simulink model "FOC_Motor_Control"  (R2020b)
settings: Solver=FixedStepDiscrete  StartTime=0.0  StopTime=10.0  FixedStep=Fixed_Step_Size  RelTol=1e-3
values from neighbouring files (symbols this model uses):
  Angle = 1.0    [Hall_HSMO_FOC_Data.sldd]    (also in Hall_SMO_FOC_Data.sldd)
  Cosine_table = 1.0 0.99999529 0.99999058 0.99998587 0.99998116 0.99996704 0.99995291 0.99993885 0.99992472 0.99990118 0.99987763 0.99985409 0.9998306 0.99979764 0.99976468 0.99973178 0.99969882 0.99965644 0.99961412 0.99957174 0.99952942 0.99947762 0.99942589 0.99937415 0.99932235 0.9992612 0.99920005 0.99913889 0.99907768 0.99900717 0.99893659 0.99886602 0.99879545 0.99871546 0.99863547 0.99855554 0.99847555 0.    [Hall_HSMO_FOC_Data.sldd]    (also in Hall_SMO_FOC_Data.sldd)
  Flux = 0.0109    [G474_FOC_HSMO.sldd]    (also in Hall_HSMO_FOC_Data.sldd = 0.00529276
  HaLL_AngleShift = -0.25    [Hall_HSMO_FOC_Data.sldd]    (also in Hall_SMO_FOC_Data.sldd)
  HaLL_Sector1 = 5.236    [Hall_HSMO_FOC_Data.sldd]    (also in Hall_SMO_FOC_Data.sldd)
  HaLL_Sector2 = 1.0472    [Hall_HSMO_FOC_Data.sldd]    (also in Hall_SMO_FOC_Data.sldd)
  HaLL_Sector3 = 0.0    [Hall_HSMO_FOC_Data.sldd]    (also in Hall_SMO_FOC_Data.sldd)
  HaLL_Sector4 = 3.1415    [Hall_HSMO_FOC_Data.sldd]    (also in Hall_SMO_FOC_Data.sldd)
  HaLL_Sector5 = 4.1888    [Hall_HSMO_FOC_Data.sldd]    (also in Hall_SMO_FOC_Data.sldd)
  HaLL_Sector6 = 2.0944    [Hall_HSMO_FOC_Data.sldd]    (also in Hall_SMO_FOC_Data.sldd)
  HaLL_Timer_T = 1.0E-5    [Hall_HSMO_FOC_Data.sldd]    (also in Hall_SMO_FOC_Data.sldd)
  ID_Ki = 450.0    [Hall_HSMO_FOC_Data.sldd]    (also in Hall_SMO_FOC_Data.sldd = 0.8
  ID_Kp = 0.4    [Hall_HSMO_FOC_Data.sldd]    (also in Hall_SMO_FOC_Data.sldd = 3.2
  IQ_Ki = 450.0    [Hall_HSMO_FOC_Data.sldd]    (also in Hall_SMO_FOC_Data.sldd = 0.32
  IQ_Kp = 0.45    [Hall_HSMO_FOC_Data.sldd]    (also in Hall_SMO_FOC_Data.sldd = 3.3
  LADRC_b0 = 80000.0    [Hall_HSMO_FOC_Data.sldd]    (also in Hall_SMO_FOC_Data.sldd)
  LADRC_Omega_c = 80.0    [Hall_HSMO_FOC_Data.sldd]    (also in Hall_SMO_FOC_Data.sldd)
  Ld = 0.000195185    [G474_FOC_HSMO.sldd]    (also in Hall_HSMO_FOC_Data.sldd = 0.0004
  Lq = 0.000195185    [G474_FOC_HSMO.sldd]    (also in Hall_HSMO_FOC_Data.sldd = 0.00045
  OPL_Speed = 800.0    [Hall_HSMO_FOC_Data.sldd]
  OPL_Time = 5.0    [Hall_HSMO_FOC_Data.sldd]
  OPL_Torque = 3.0    [Hall_HSMO_FOC_Data.sldd]
  Over_modulation = 0.0    [Hall_HSMO_FOC_Data.sldd]    (also in Hall_SMO_FOC_Data.sldd)
  Pole_Pairs = 2.0    [Hall_HSMO_FOC_Data.sldd]    (also in Hall_SMO_FOC_Data.sldd)
  PWM_Frequency = 10000.0    [Hall_HSMO_FOC_Data.sldd]    (also in Hall_SMO_FOC_Data.sldd)
  R = 0.405    [Hall_HSMO_FOC_Data.sldd]    (also in Hall_SMO_FOC_Data.sldd = 0.4
  Sine_table = 0.0 0.0015339879 0.0030679768 0.0046019657 0.0061359555 0.0076698866 0.0092038177 0.010737749 0.012271681 0.013805497 0.015339312 0.016873131 0.018406944 0.019940587 0.021474229 0.023007872 0.024541514 0.026074925 0.027608337 0.029141748 0.03067516 0.032208283 0.033741407 0.035274528 0.036807653 0.038340431 0.039873205 0.04140598 0.042938754 0.04447113 0.046003502 0.047535874 0.049068246 0.0506001    [Hall_HSMO_FOC_Data.sldd]    (also in Hall_SMO_FOC_Data.sldd)
  SMO_K = 0.5    [Hall_HSMO_FOC_Data.sldd]    (also in Hall_SMO_FOC_Data.sldd)
  SMO_M = 0.15    [Hall_HSMO_FOC_Data.sldd]    (also in Hall_SMO_FOC_Data.sldd)
  SMO_PLL_W = 50.0    [Hall_HSMO_FOC_Data.sldd]    (also in Hall_SMO_FOC_Data.sldd)
  SMO_Theta_Enable = 0.0    [Hall_HSMO_FOC_Data.sldd]    (also in Hall_SMO_FOC_Data.sldd = 1.0
  Speed_Ki = 0.633    [Hall_HSMO_FOC_Data.sldd]    (also in Hall_SMO_FOC_Data.sldd)
  Speed_Kp = 0.0867    [Hall_HSMO_FOC_Data.sldd]    (also in Hall_SMO_FOC_Data.sldd = 0.0267
  Speed_PI_OutputMax = 6.0    [Hall_HSMO_FOC_Data.sldd]    (also in Hall_SMO_FOC_Data.sldd = 5.0
  Speed_PI_OutputMin = -6.0    [Hall_HSMO_FOC_Data.sldd]    (also in Hall_SMO_FOC_Data.sldd = -5.0
  SpeedFilter_Fn = 0.3    [Hall_HSMO_FOC_Data.sldd]    (also in Hall_SMO_FOC_Data.sldd)
  TorqueMode = 0.0    [Hall_HSMO_FOC_Data.sldd]    (also in Hall_SMO_FOC_Data.sldd)
undefined symbols (not defined in the file or in its folder): DiscIntNeverNeededParam, inverter, magnitude, SVPWM
libraries: simulink x6, pid_lib x1
(part 2 of 3)

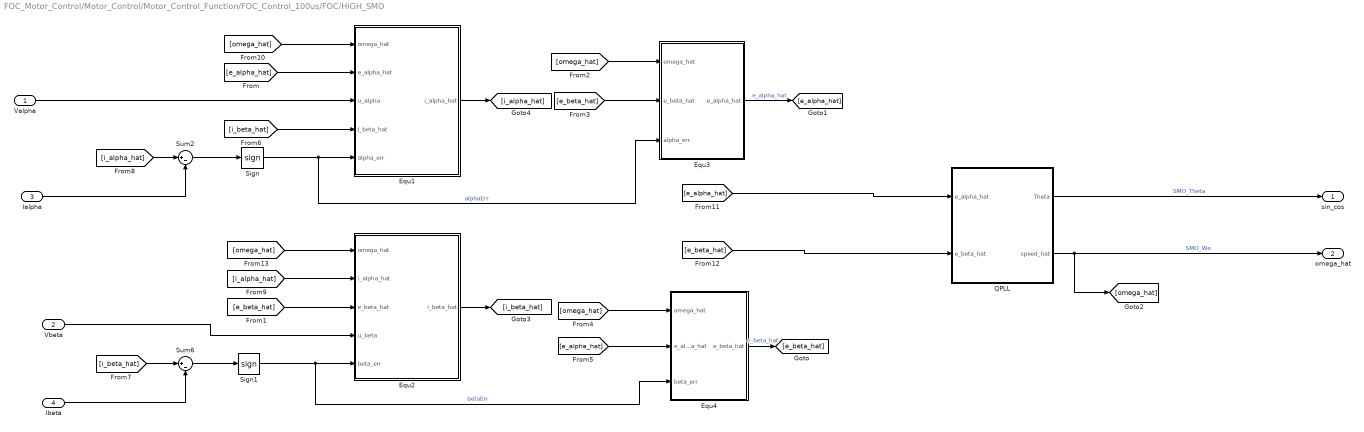
== system FOC_Motor_Control/Motor_Control/Motor_Control_Function/FOC_Control_100us/FOC/HIGH_SMO ==
  Valpha : Inport
  Vbeta : Inport  Port=2
  Ialpha : Inport  Port=3
  Ibeta : Inport  Port=4
  Equ1 : Subsystem
  Equ2 : Subsystem
  Equ3 : Subsystem
  Equ4 : Subsystem
  QPLL : Subsystem
  Sign : Signum
  Sign1 : Signum
  Sum2 : Sum  Inputs=|+-
  Sum6 : Sum  Inputs=|+-
  sin_cos : Outport
  omega_hat : Outport  Port=2
  wires:
  Sum6/1 -> Sign1/1
  Sum2/1 -> Sign/1
  Sign/1 -> Equ3/3(alpha_err), Equ1/5(alpha_err)  "alphaErr"
  Ialpha/1 -> Sum2/2
  Sign1/1 -> Equ4/3(beta_err), Equ2/5(beta_err)  "betaErr"
  Ibeta/1 -> Sum6/2
  Equ1/1(i_alpha_hat) -> [i_alpha_hat]
  [e_alpha_hat] -> Equ1/2(e_alpha_hat)
  Valpha/1 -> Equ1/3(u_alpha)
  [e_beta_hat] -> Equ2/3(e_beta_hat)
  Vbeta/1 -> Equ2/4(u_beta)
  Equ2/1(i_beta_hat) -> [i_beta_hat]
  [i_beta_hat] -> Equ1/4(I_beta_hat)
  [i_beta_hat] -> Sum6/1
  [i_alpha_hat] -> Sum2/1
  [i_alpha_hat] -> Equ2/2(i_alpha_hat)
  [omega_hat] -> Equ3/1(omega_hat)
  [e_beta_hat] -> Equ3/2(e_beta_hat)
  [omega_hat] -> Equ4/1(omega_hat)
  [e_alpha_hat] -> Equ4/2(e_alpha_hat)
  [omega_hat] -> Equ1/1(omega_hat)
  Equ4/1(e_beta_hat) -> [e_beta_hat]  "e_beta_hat"
  Equ3/1(e_alpha_hat) -> [e_alpha_hat]  "e_alpha_hat"
  [e_alpha_hat] -> QPLL/1(e_alpha_hat)
  [e_beta_hat] -> QPLL/2(e_beta_hat)
  QPLL/2(speed_hat) -> [omega_hat], omega_hat/1  "SMO_We"
  QPLL/1(Theta) -> sin_cos/1  "SMO_Theta"
  [omega_hat] -> Equ2/1(omega_hat)

== system FOC_Motor_Control/Motor_Control/Motor_Control_Function/FOC_Control_100us/FOC/Hall_Angle ==
  Hall_Angle : Inport
  Action Port : ActionPort  ActionPortLabel=elseif(u1==0)
  Out1 : Outport
  wires:
  Hall_Angle/1 -> Out1/1

== system FOC_Motor_Control/Motor_Control/Motor_Control_Function/FOC_Control_100us/FOC/Inverse_Park_Transform ==
  D : Inport
  Q : Inport  Port=2
  Sin_Coefficient : Inport  Port=3
  Cos_Coefficient : Inport  Port=4
  Add1 : Sum  Inputs=+-  OutDataTypeStr=Inherit: Same as first input
  Add2 : Sum  OutDataTypeStr=Inherit: Same as first input
  Cos_Coefficient1 : InportShadow  Port=4
  Product{1..4} (4 alike) : Product  RndMeth=Simplest  OutDataTypeStr=Inherit: Same as first input
  Sin_Coefficient1 : InportShadow  Port=3
  Alpha : Outport  VectorParamsAs1DForOutWhenUnconnected=off
  Beta : Outport  Port=2  VectorParamsAs1DForOutWhenUnconnected=off
  wires:
  Product3/1 -> Add2/1
  Product4/1 -> Add2/2
  Product1/1 -> Add1/1
  Product2/1 -> Add1/2
  Cos_Coefficient1/1 -> Product4/2
  Sin_Coefficient/1 -> Product2/2
  D/1 -> Product3/1, Product1/1
  Q/1 -> Product2/1, Product4/1
  Sin_Coefficient1/1 -> Product3/2
  Cos_Coefficient/1 -> Product1/2
  Add1/1 -> Alpha/1
  Add2/1 -> Beta/1

== system FOC_Motor_Control/Motor_Control/Motor_Control_Function/FOC_Control_100us/FOC/LPF ==
  u : Inport
  Add : Sum  Inputs=+-
  Add1 : Sum
  Constant1 : Constant  Value=SpeedFilter_Fn  OutDataTypeStr=single
  Divide1 : Product  Inputs=**
  Unit Delay : UnitDelay  SampleTime=-1  HasFrameUpgradeWarning=on
  y : Outport
  wires:
  Constant1/1 -> Divide1/1
  u/1 -> Add/1
  Add/1 -> Divide1/2
  Divide1/1 -> Add1/1
  Unit Delay/1 -> Add/2, Add1/2
  Add1/1 -> Unit Delay/1, y/1

== system FOC_Motor_Control/Motor_Control/Motor_Control_Function/FOC_Control_100us/FOC/Obs_Angle ==
  Obs_Angle : Inport
  Action Port : ActionPort  ActionPortLabel=if(u1==1)
  Out1 : Outport
  wires:
  Obs_Angle/1 -> Out1/1

== system FOC_Motor_Control/Motor_Control/Motor_Control_Function/FOC_Control_100us/FOC/OpenLoop ==
  OPL_Speed : Inport
  OPL_Torque : Inport  Port=2
  OPL_Time : Inport  Port=3
  Action Port : ActionPort  ActionPortLabel=case [ 1 ]:
  2pi2 : Constant  Value=2*pi  OutDataTypeStr=single
  Discrete-Time Integrator1 : DiscreteIntegrator  SampleTime=-1  ICPrevOutput=DiscIntNeverNeededParam  ICPrevScaledInput=DiscIntNeverNeededParam
  Discrete-Time Integrator2 : DiscreteIntegrator  SampleTime=-1  ICPrevOutput=DiscIntNeverNeededParam  ICPrevScaledInput=DiscIntNeverNeededParam
  Mod2 : Math  Operator=mod  SaturateOnIntegerOverflow=on
  Product : Product
  Scope : Scope
  Scope1 : Scope
  We : Gain  Gain=Pole_Pairs*2*pi/60  OutDataTypeStr=single  ParamDataTypeStr=Inherit: Same as input
  Force_Angle : Outport
  OPL_Torque_Com : Outport  Port=2
  wires:
  OPL_Speed/1 -> Product/1
  Product/1 -> Discrete-Time Integrator2/1
  Discrete-Time Integrator1/1 -> Mod2/1
  Discrete-Time Integrator2/1 -> Scope/1, We/1
  We/1 -> Discrete-Time Integrator1/1  "Delta_Theta"
  Mod2/1 -> Force_Angle/1, Scope1/1
  OPL_Torque/1 -> OPL_Torque_Com/1
  OPL_Time/1 -> Product/2
  2pi2/1 -> Mod2/2

== system FOC_Motor_Control/Motor_Control/Motor_Control_Function/FOC_Control_100us/FOC/Park_Transform ==
  Alpha : Inport
  Beta : Inport  Port=2
  Sin_Coefficient : Inport  Port=3
  Cos_Coefficient : Inport  Port=4
  Add1 : Sum  OutDataTypeStr=Inherit: Same as first input
  Add2 : Sum  Inputs=-+  OutDataTypeStr=Inherit: Same as first input
  Alpha1 : InportShadow
  Beta1 : InportShadow  Port=2
  Cos_Coefficient1 : InportShadow  Port=4
  Produc3t : Product  RndMeth=Simplest  OutDataTypeStr=Inherit: Same as first input
  Product1 : Product  RndMeth=Simplest  OutDataTypeStr=Inherit: Same as first input
  Product2 : Product  RndMeth=Simplest  OutDataTypeStr=Inherit: Same as first input
  Product4 : Product  RndMeth=Simplest  OutDataTypeStr=Inherit: Same as first input
  Sin_Coefficient1 : InportShadow  Port=3
  D : Outport  VectorParamsAs1DForOutWhenUnconnected=off
  Q : Outport  Port=2  VectorParamsAs1DForOutWhenUnconnected=off
  wires:
  Produc3t/1 -> Add2/1
  Product4/1 -> Add2/2
  Product1/1 -> Add1/1
  Product2/1 -> Add1/2
  Alpha1/1 -> Produc3t/1
  Sin_Coefficient1/1 -> Produc3t/2
  Cos_Coefficient1/1 -> Product4/2
  Beta1/1 -> Product4/1
  Alpha/1 -> Product1/1
  Cos_Coefficient/1 -> Product1/2
  Beta/1 -> Product2/1
  Sin_Coefficient/1 -> Product2/2
  Add1/1 -> D/1
  Add2/1 -> Q/1

== system FOC_Motor_Control/Motor_Control/Motor_Control_Function/FOC_Control_100us/FOC/Q_Current_PI ==
  Reset : Inport
  Bus_voltage : Inport  Port=2
  Current_Command : Inport  Port=3
  Current_Measured : Inport  Port=4
  Add2 : Sum  Inputs=|+-
  IQ_Control : Subsystem
  Vq_voltage : Outport  VectorParamsAs1DForOutWhenUnconnected=off
  wires:
  Current_Command/1 -> Add2/1
  Current_Measured/1 -> Add2/2
  Add2/1 -> IQ_Control/3(Err)  "currentControlError"
  Reset/1 -> IQ_Control/1(Reset)
  Bus_voltage/1 -> IQ_Control/2(Bus_voltage)
  IQ_Control/1(PI_Out) -> Vq_voltage/1

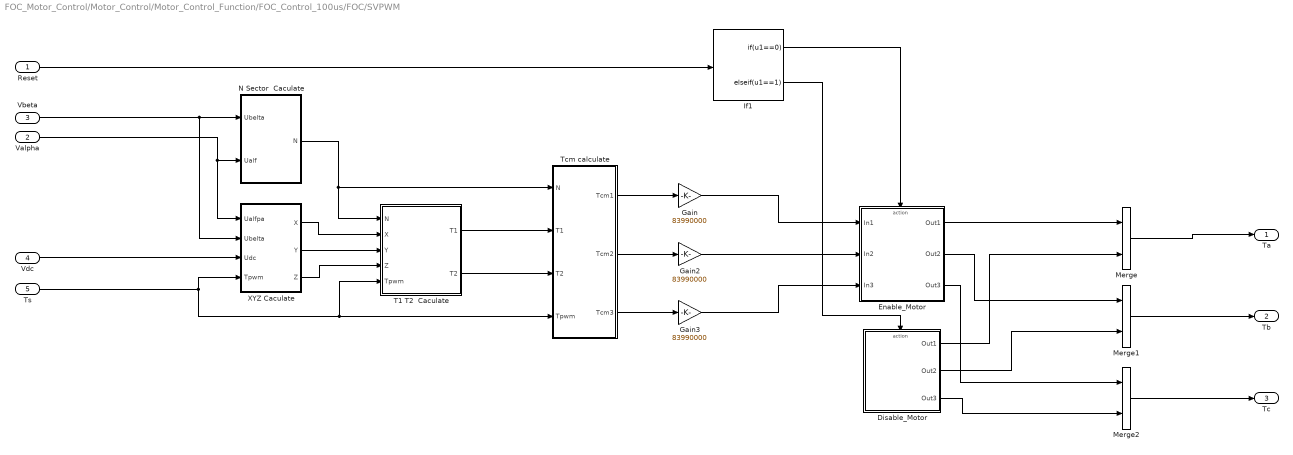
== system FOC_Motor_Control/Motor_Control/Motor_Control_Function/FOC_Control_100us/FOC/SVPWM ==
  Reset : Inport
  Valpha : Inport  Port=2
  Vbeta : Inport  Port=3
  Vdc : Inport  Port=4
  Ts : Inport  Port=5
  Disable_Motor : Subsystem  TreatAsAtomicUnit=on
  Enable_Motor : Subsystem  TreatAsAtomicUnit=on
  Gain : Gain  Gain=83990000
  Gain2 : Gain  Gain=83990000
  Gain3 : Gain  Gain=83990000
  If1 : If  IfExpression=u1==0  ElseIfExpressions=u1==1  ShowElse=off
  Merge : Merge
  Merge1 : Merge
  Merge2 : Merge
  N Sector  Caculate : Subsystem  TreatAsAtomicUnit=on
  T1 T2  Caculate : Subsystem  TreatAsAtomicUnit=on
  Tcm calculate : Subsystem  TreatAsAtomicUnit=on
  XYZ Caculate : Subsystem  TreatAsAtomicUnit=on
  Ta : Outport
  Tb : Outport  Port=2
  Tc : Outport  Port=3
  wires:
  T1 T2  Caculate/2(T2) -> Tcm calculate/3(T2)
  XYZ Caculate/1(X) -> T1 T2  Caculate/2(X)
  N Sector  Caculate/1(N) -> T1 T2  Caculate/1(N), Tcm calculate/1(N)
  Vdc/1 -> XYZ Caculate/3(Udc)
  T1 T2  Caculate/1(T1) -> Tcm calculate/2(T1)
  XYZ Caculate/3(Z) -> T1 T2  Caculate/4(Z)
  XYZ Caculate/2(Y) -> T1 T2  Caculate/3(Y)
  Valpha/1 -> N Sector  Caculate/2(Ualf), XYZ Caculate/1(Ualfpa)
  Vbeta/1 -> N Sector  Caculate/1(Ubelta), XYZ Caculate/2(Ubelta)
  Ts/1 -> T1 T2  Caculate/5(Tpwm), Tcm calculate/4(Tpwm), XYZ Caculate/4(Tpwm)
  Gain/1 -> Enable_Motor/1(In1)
  Gain2/1 -> Enable_Motor/2(In2)
  Reset/1 -> If1/1
  If1/1 -> Enable_Motor/Action
  If1/2 -> Disable_Motor/Action
  Gain3/1 -> Enable_Motor/3(In3)
  Enable_Motor/1(Out1) -> Merge/1
  Disable_Motor/1(Out1) -> Merge/2
  Enable_Motor/2(Out2) -> Merge1/1
  Disable_Motor/2(Out2) -> Merge1/2
  Enable_Motor/3(Out3) -> Merge2/1
  Disable_Motor/3(Out3) -> Merge2/2
  Merge/1 -> Ta/1
  Merge1/1 -> Tb/1
  Merge2/1 -> Tc/1
  Tcm calculate/1(Tcm1) -> Gain/1
  Tcm calculate/2(Tcm2) -> Gain2/1
  Tcm calculate/3(Tcm3) -> Gain3/1

== system FOC_Motor_Control/Motor_Control/Motor_Control_Function/FOC_Control_100us/FOC/Sine_Cosine ==
  note: Sine Cosine Coefficients
  P : Inport
  Cosine : Lookup_n-D  NumberOfTableDimensions=1  LookupTableObject=''  BreakpointsForDimension1=[0:2*pi/4095:2*pi]  BreakpointsForDimension1FirstPoint=10  BreakpointsForDimension2FirstPoint=10  BreakpointsForDimension1Spacing=12  BreakpointsForDimension2Spacing=12  IndexSearchMethod=Evenly spaced points  Table=Cosine_table  InterpMethod=Flat  DiagnosticForOutOfRangeInput=Error  InternalRulePriority=Speed  RndMeth=Simplest  InputSameDT=on
  Saturation : Saturate  UpperLimit=2*pi-0.0001  LowerLimit=0+0.0001
  Scope : Scope  NumInputPorts=2
  Sine : Lookup_n-D  NumberOfTableDimensions=1  LookupTableObject=''  BreakpointsForDimension1=[0:2*pi/4095:2*pi]  BreakpointsForDimension1FirstPoint=10  BreakpointsForDimension2FirstPoint=10  BreakpointsForDimension1Spacing=12  BreakpointsForDimension2Spacing=12  IndexSearchMethod=Evenly spaced points  Table=Sine_table  InterpMethod=Flat  DiagnosticForOutOfRangeInput=Error  InternalRulePriority=Speed  RndMeth=Simplest  InputSameDT=on
  Sin : Outport  VectorParamsAs1DForOutWhenUnconnected=off
  Cos : Outport  Port=2  VectorParamsAs1DForOutWhenUnconnected=off
  wires:
  P/1 -> Saturation/1  "position"
  Sine/1 -> Scope/1, Sin/1
  Cosine/1 -> Scope/2, Cos/1
  Saturation/1 -> Cosine/1, Sine/1

== system FOC_Motor_Control/Motor_Control/Motor_Control_Function/FOC_Control_100us/FOC/Subsystem ==
  In1 : Inport
  In2 : Inport  Port=2
  Action Port : ActionPort  ActionPortLabel=case [ 2 ]:
  Out1 : Outport
  Out2 : Outport  Port=2
  wires:
  In1/1 -> Out1/1
  In2/1 -> Out2/1

== system FOC_Motor_Control/Motor_Control/Motor_Control_Function/Angle_Speed_100us/SpeedAndAngle/ACC_OMG/LPF ==
  u : Inport
  Add : Sum  Inputs=+-
  Add1 : Sum
  Constant1 : Constant  Value=SpeedFilter_Fn  OutDataTypeStr=single
  Divide1 : Product  Inputs=**
  Unit Delay : UnitDelay  SampleTime=-1  HasFrameUpgradeWarning=on
  y : Outport
  wires:
  Constant1/1 -> Divide1/1
  u/1 -> Add/1
  Add/1 -> Divide1/2
  Divide1/1 -> Add1/1
  Unit Delay/1 -> Add/2, Add1/2
  Add1/1 -> Unit Delay/1, y/1

== system FOC_Motor_Control/Motor_Control/Motor_Control_Function/Angle_Speed_100us/SpeedAndAngle/ACC_OMG/Six_point ==
  In1 : Inport
  Merge2 : Merge  Inputs=6
  Scope : Scope  NumInputPorts=2
  Sector_1 : Subsystem
  Sector_2 : Subsystem
  Sector_3 : Subsystem
  Sector_4 : Subsystem
  Sector_5 : Subsystem
  Sector_6 : Subsystem
  Switch Case2 : SwitchCase  CaseConditions={1,2,3,4,5,6}  ShowDefaultCase=off
  Out1 : Outport
  wires:
  Sector_4/1(Angle_0) -> Merge2/4
  Switch Case2/5 -> Sector_5/Action
  Sector_6/1(Angle_0) -> Merge2/6
  Sector_5/1(Angle_0) -> Merge2/5
  Switch Case2/6 -> Sector_6/Action
  Switch Case2/3 -> Sector_3/Action
  Switch Case2/4 -> Sector_4/Action
  Sector_1/1(Angle_0) -> Merge2/1
  Switch Case2/2 -> Sector_2/Action
  In1/1 -> Scope/1, Switch Case2/1
  Sector_3/1(Angle_0) -> Merge2/3
  Switch Case2/1 -> Sector_1/Action
  Sector_2/1(Angle_0) -> Merge2/2
  Merge2/1 -> Scope/2, Out1/1

== system FOC_Motor_Control/Motor_Control/Motor_Control_Function/Angle_Speed_100us/SpeedAndAngle/ADC_IRQ/HallAngle_calibration ==
  Angle_input : Inport
  Angle_offset : Constant  Value=HaLL_AngleShift
  If Action Subsystem1 : Subsystem  TreatAsAtomicUnit=on
  If Action Subsystem2 : Subsystem  TreatAsAtomicUnit=on
  If Action Subsystem3 : Subsystem  TreatAsAtomicUnit=on
  If1 : If  IfExpression=u1 > 6.283185307  ElseIfExpressions=u1<0
  Merge1 : Merge  Inputs=3
  Subtract1 : Sum
  Angle_output : Outport
  wires:
  Angle_input/1 -> Subtract1/1
  Angle_offset/1 -> Subtract1/2  "Control_ModeCommand"
  If1/1 -> If Action Subsystem2/Action
  If1/3 -> If Action Subsystem1/Action
  If Action Subsystem2/1(Out1) -> Merge1/1
  Subtract1/1 -> If Action Subsystem3/1(In1), If Action Subsystem1/1(In1), If Action Subsystem2/1(In1), If1/1
  If Action Subsystem1/1(Out1) -> Merge1/3
  If Action Subsystem3/1(Out1) -> Merge1/2
  If1/2 -> If Action Subsystem3/Action
  Merge1/1 -> Angle_output/1

== system FOC_Motor_Control/Motor_Control/Motor_Control_Function/Angle_Speed_100us/Speed_Resolver/Speed_cacl/LPF ==
  u : Inport
  Add : Sum  Inputs=+-
  Add1 : Sum
  Constant1 : Constant  Value=SpeedFilter_Fn  OutDataTypeStr=single
  Divide1 : Product  Inputs=**
  Unit Delay : UnitDelay  SampleTime=-1  HasFrameUpgradeWarning=on
  y : Outport
  wires:
  Constant1/1 -> Divide1/1
  u/1 -> Add/1
  Add/1 -> Divide1/2
  Divide1/1 -> Add1/1
  Unit Delay/1 -> Add/2, Add1/2
  Add1/1 -> Unit Delay/1, y/1

== system FOC_Motor_Control/Motor_Control/Motor_Control_Function/Control_Command_2ms/Control_Command_2ms/Speed_PI/SpeedLoop ==
  CMD_RPM : Inport  OutDataTypeStr=single
  FdkRPM : Inport  Port=2  OutDataTypeStr=single
  Reset : Inport  Port=3
  Constant : Constant  Value=LADRC_b0  OutDataTypeStr=single  SampleTime=-1
  Divide : Product  Inputs=*/  OutDataTypeStr=single
  LESO : Subsystem
  Saturation : Saturate  UpperLimit=Speed_PI_OutputMax  LowerLimit=Speed_PI_OutputMin  OutDataTypeStr=single
  Sum : Sum  Inputs=|+-  OutDataTypeStr=single
  Sum1 : Sum  Inputs=|+-  OutDataTypeStr=single
  Unit Delay : UnitDelay  SampleTime=-1  HasFrameUpgradeWarning=on
  omega_c : Gain  Gain=LADRC_Omega_c  OutDataTypeStr=single
  RefIq : Outport  OutDataTypeStr=single
  wires:
  Saturation/1 -> RefIq/1, Unit Delay/1
  Constant/1 -> Divide/2
  Divide/1 -> Saturation/1
  LESO/2(f_hat) -> Sum1/2
  FdkRPM/1 -> LESO/1(FbkSpd)  "FdkRPM"
  LESO/1(omega_r_hat) -> Sum/2
  Sum1/1 -> Divide/1
  omega_c/1 -> Sum1/1
  Sum/1 -> omega_c/1
  CMD_RPM/1 -> Sum/1  "CMD_RPM"
  Unit Delay/1 -> LESO/2(iq)
  Reset/1 -> LESO/3(Reset)

== system FOC_Motor_Control/Motor_Control/Motor_Control_Function/Control_Command_2ms/Control_Command_2ms/Speed_PI/Speed_PI ==
  Ref : Inport
  Fdk : Inport  Port=2
  Reset : Inport  Port=3
  Speed_Control : Subsystem
  Sum : Sum  Inputs=|+-
  PI_out : Outport  VectorParamsAs1DForOutWhenUnconnected=off
  wires:
  Speed_Control/1(PI_Out) -> PI_out/1
  Reset/1 -> Speed_Control/2(Reset)
  Ref/1 -> Sum/1
  Sum/1 -> Speed_Control/1(Err)
  Fdk/1 -> Sum/2

== system FOC_Motor_Control/Motor_Control/Motor_Control_Function/FOC_Control_100us/FOC/Clarke_Transform/Clark1 ==
  Iabc : Inport
  Add : Sum  Inputs=+--
  Add1 : Sum  Inputs=+-
  Demux : Demux  Outputs=3
  Gain : Gain  Gain=0.5
  Gain1 : Gain  Gain=0.5
  Gain2 : Gain  Gain=sqrt(2/3)
  Gain3 : Gain  Gain=sqrt(3)/2
  Gain4 : Gain  Gain=sqrt(3)/2
  Gain5 : Gain  Gain=sqrt(2/3)
  Ialpha : Outport  VectorParamsAs1DForOutWhenUnconnected=off
  Ibeta : Outport  Port=2  VectorParamsAs1DForOutWhenUnconnected=off
  wires:
  Iabc/1 -> Demux/1
  Demux/1 -> Add/1
  Gain/1 -> Add/2
  Demux/2 -> Gain3/1, Gain/1
  Gain1/1 -> Add/3
  Demux/3 -> Gain4/1, Gain1/1
  Add/1 -> Gain2/1
  Gain2/1 -> Ialpha/1
  Gain3/1 -> Add1/1
  Gain4/1 -> Add1/2
  Add1/1 -> Gain5/1
  Gain5/1 -> Ibeta/1

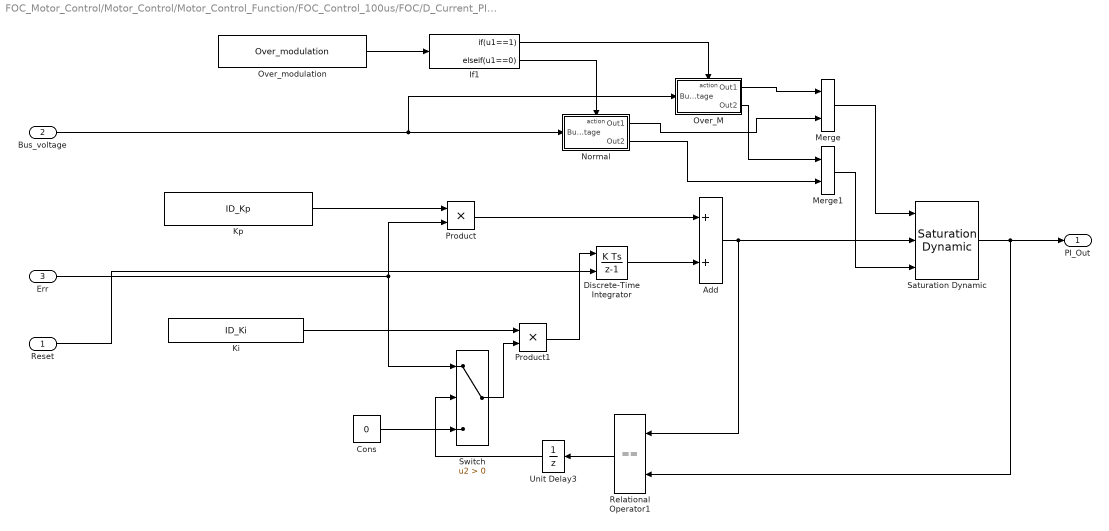
== system FOC_Motor_Control/Motor_Control/Motor_Control_Function/FOC_Control_100us/FOC/D_Current_PI/ID_Control ==
  Reset : Inport
  Bus_voltage : Inport  Port=2
  Err : Inport  Port=3
  Add : Sum
  Cons : Constant  Value=0  OutDataTypeStr=single
  Discrete-Time Integrator : DiscreteIntegrator  ExternalReset=level  SampleTime=-1  ICPrevOutput=DiscIntNeverNeededParam  ICPrevScaledInput=DiscIntNeverNeededParam
  If1 : If  IfExpression=u1==1  ElseIfExpressions=u1==0  ShowElse=off
  Ki : Constant  Value=ID_Ki  OutDataTypeStr=single
  Kp : Constant  Value=ID_Kp  OutDataTypeStr=single
  Merge : Merge
  Merge1 : Merge
  Normal : Subsystem  TreatAsAtomicUnit=on
  Over_M : Subsystem  TreatAsAtomicUnit=on
  Over_modulation : Constant  Value=Over_modulation  OutDataTypeStr=boolean
  Product : Product
  Product1 : Product
  Relational Operator1 : RelationalOperator  Operator===  OutDataTypeStr=boolean  RndMeth=Simplest
  Saturation Dynamic : simulink/Discontinuities/Saturation Dynamic  OutMin=[]  OutMax=[]  OutDataTypeStr=Inherit: Same as second input  OutDataType=fixdt(1, 16)  OutScaling=2^-10  DoSatur=off
  Switch : Switch  Criteria=u2 > Threshold
  Unit Delay3 : UnitDelay  SampleTime=-1  HasFrameUpgradeWarning=on
  PI_Out : Outport
  wires:
  Kp/1 -> Product/1
  Err/1 -> Product/2, Switch/1
  Switch/1 -> Product1/2
  Product1/1 -> Discrete-Time Integrator/1
  Product/1 -> Add/1
  Add/1 -> Saturation Dynamic/2, Relational Operator1/1
  Saturation Dynamic/1 -> Relational Operator1/2, PI_Out/1
  Cons/1 -> Switch/3
  Discrete-Time Integrator/1 -> Add/2
  Relational Operator1/1 -> Unit Delay3/1
  Ki/1 -> Product1/1
  Unit Delay3/1 -> Switch/2
  Reset/1 -> Discrete-Time Integrator/2
  Over_modulation/1 -> If1/1
  If1/2 -> Normal/Action
  If1/1 -> Over_M/Action
  Bus_voltage/1 -> Over_M/1(Bus_voltage), Normal/1(Bus_voltage)
  Over_M/1(Out1) -> Merge/1
  Normal/1(Out1) -> Merge/2
  Over_M/2(Out2) -> Merge1/1
  Normal/2(Out2) -> Merge1/2
  Merge/1 -> Saturation Dynamic/1
  Merge1/1 -> Saturation Dynamic/3

== system FOC_Motor_Control/Motor_Control/Motor_Control_Function/FOC_Control_100us/FOC/HIGH_SMO/Equ1 ==
  note: GainK/Ld
  note: R/Ld
  note: (Ld-Lq)/Ld
  note: 1/Ld
  note: 1/Ld
  omega_hat : Inport
  e_alpha_hat : Inport  Port=2
  u_alpha : Inport  Port=3
  I_beta_hat : Inport  Port=4
  alpha_err : Inport  Port=5
  Add : Sum  Inputs=---+-
  Gain : Gain  Gain=R/Ld
  Gain1 : Gain  Gain=(Ld-Lq)/Ld
  Gain17 : Gain  Gain=1/Ld
  Gain2 : Gain  Gain=1/Ld
  Gain4 : Gain  Gain=SMO_K/Ld
  Integrator : DiscreteIntegrator  IntegratorMethod=Integration: Backward Euler  SampleTime=-1  ICPrevOutput=DiscIntNeverNeededParam  ICPrevScaledInput=DiscIntNeverNeededParam  mask(DiscretizedDiscreteIntegrator){}
      mask init:
      | %tustin
  Product : Product
  Unit Delay : UnitDelay  SampleTime=-1  HasFrameUpgradeWarning=on
  i_alpha_hat : Outport
  wires:
  Gain1/1 -> Add/2
  Gain4/1 -> Add/5
  Product/1 -> Gain1/1
  Add/1 -> Integrator/1
  I_beta_hat/1 -> Product/1
  Unit Delay/1 -> [i_alpha_hat], i_alpha_hat/1
  Gain/1 -> Add/1
  u_alpha/1 -> Gain2/1
  Gain2/1 -> Add/4
  Integrator/1 -> Unit Delay/1
  omega_hat/1 -> Product/2
  Gain17/1 -> Add/3
  e_alpha_hat/1 -> Gain17/1
  alpha_err/1 -> Gain4/1
  [i_alpha_hat] -> Gain/1

== system FOC_Motor_Control/Motor_Control/Motor_Control_Function/FOC_Control_100us/FOC/HIGH_SMO/Equ2 ==
  note: R/Ld
  note: (Ld-Lq)/Ld
  note: 1/Ld
  note: 1/Ld
  note: GainK/Ld
  omega_hat : Inport
  i_alpha_hat : Inport  Port=2
  e_beta_hat : Inport  Port=3
  u_beta : Inport  Port=4
  beta_err : Inport  Port=5
  Add1 : Sum  Inputs=+--+-
  Gain3 : Gain  Gain=1/Ld
  Gain5 : Gain  Gain=1/Ld
  Gain6 : Gain  Gain=SMO_K/Ld
  Gain7 : Gain  Gain=(Ld-Lq)/Ld
  Gain8 : Gain  Gain=R/Ld
  Integrator1 : DiscreteIntegrator  IntegratorMethod=Integration: Backward Euler  SampleTime=-1  ICPrevOutput=DiscIntNeverNeededParam  ICPrevScaledInput=DiscIntNeverNeededParam  mask(DiscretizedDiscreteIntegrator){}
      mask init:
      | %tustin
  Product1 : Product
  Unit Delay1 : UnitDelay  SampleTime=-1  HasFrameUpgradeWarning=on
  i_beta_hat : Outport
  wires:
  Gain8/1 -> Add1/2
  u_beta/1 -> Gain5/1
  Add1/1 -> Integrator1/1
  Gain3/1 -> Add1/3
  i_alpha_hat/1 -> Product1/1
  Gain5/1 -> Add1/4
  Gain6/1 -> Add1/5
  Integrator1/1 -> Unit Delay1/1
  Product1/1 -> Gain7/1
  Gain7/1 -> Add1/1
  beta_err/1 -> Gain6/1
  e_beta_hat/1 -> Gain3/1
  Unit Delay1/1 -> [I_beta_hat], i_beta_hat/1
  omega_hat/1 -> Product1/2
  [I_beta_hat] -> Gain8/1

== system FOC_Motor_Control/Motor_Control/Motor_Control_Function/FOC_Control_100us/FOC/HIGH_SMO/Equ3 ==
  omega_hat : Inport
  e_beta_hat : Inport  Port=2
  alpha_err : Inport  Port=3
  Add2 : Sum  Inputs=-+
  Gain9 : Gain  Gain=SMO_M/Ld
  Integrator2 : DiscreteIntegrator  IntegratorMethod=Integration: Backward Euler  SampleTime=-1  ICPrevOutput=DiscIntNeverNeededParam  ICPrevScaledInput=DiscIntNeverNeededParam  mask(DiscretizedDiscreteIntegrator){}
      mask init:
      | %tustin
  Product2 : Product
  Unit Delay2 : UnitDelay  SampleTime=-1  HasFrameUpgradeWarning=on
  e_alpha_hat : Outport
  wires:
  alpha_err/1 -> Gain9/1
  Add2/1 -> Integrator2/1
  Unit Delay2/1 -> e_alpha_hat/1
  omega_hat/1 -> Product2/1
  Product2/1 -> Add2/1
  Integrator2/1 -> Unit Delay2/1
  e_beta_hat/1 -> Product2/2
  Gain9/1 -> Add2/2

== system FOC_Motor_Control/Motor_Control/Motor_Control_Function/FOC_Control_100us/FOC/HIGH_SMO/Equ4 ==
  omega_hat : Inport
  e_alpha_hat : Inport  Port=2
  beta_err : Inport  Port=3
  Add3 : Sum
  Gain10 : Gain  Gain=SMO_K/Ld
  Integrator3 : DiscreteIntegrator  IntegratorMethod=Integration: Backward Euler  SampleTime=-1  ICPrevOutput=DiscIntNeverNeededParam  ICPrevScaledInput=DiscIntNeverNeededParam  mask(DiscretizedDiscreteIntegrator){}
      mask init:
      | %tustin
  Product3 : Product
  Unit Delay3 : UnitDelay  SampleTime=-1  HasFrameUpgradeWarning=on
  e_beta_hat : Outport
  wires:
  Integrator3/1 -> Unit Delay3/1
  Add3/1 -> Integrator3/1
  Gain10/1 -> Add3/2
  Product3/1 -> Add3/1
  beta_err/1 -> Gain10/1
  Unit Delay3/1 -> e_beta_hat/1
  omega_hat/1 -> Product3/1
  e_alpha_hat/1 -> Product3/2

== system FOC_Motor_Control/Motor_Control/Motor_Control_Function/FOC_Control_100us/FOC/HIGH_SMO/QPLL ==
  e_alpha_hat : Inport
  e_beta_hat : Inport  Port=2
  Ki : Constant  Value=SMO_PLL_W*SMO_PLL_W  OutDataTypeStr=single
  Kp : Constant  Value=2*0.707*SMO_PLL_W  OutDataTypeStr=single
  PIDTheta_Ctrl : pid_lib/PID Controller  Controller=PI  Form=Parallel  TimeDomain=Discrete-time  UseExternalTs=off  SampleTime=-1  IntegratorMethod=Forward Euler  FilterMethod=Forward Euler  ControllerParametersSource=external  P=2*0.707*SMO_PLL_W  I=SMO_PLL_W*SMO_PLL_W  D=0  UseFilter=on  N=100  TunerSelectOption=Transfer Function Based (PID Tuner App)  ZeroCross=off  InitialConditionSource=internal  InitialConditionForIntegrator=1  InitialConditionForFilter=0  DifferentiatorICPrevScaledInput=0  ExternalReset=none  TrackingMode=off  Kt=1  LimitOutput=on  SatLimitsSource=internal  UpperSaturationLimit=2*pi*500  LowerSaturationLimit=-2*pi*500  LinearizeAsGain=off  AntiWindupMode=clamping  Kb=50  POutMin=[]  POutMax=[]  IOutMin=[]  IOutMax=[]  DOutMin=[]  DOutMax=[]  NOutMin=[]  NOutMax=[]  SumOutMin=[]  SumOutMax=[]  SaturationOutDataTypeStr=Inherit: Inherit via back propagation  SaturationOutMin=[]  SaturationOutMax=[]  PParamMin=[]  PParamMax=[]  IParamMin=[]  IParamMax=[]  DParamMin=[]  DParamMax=[]  NParamMin=[]  NParamMax=[]  KbParamMin=[]  KbParamMax=[]  KtParamMin=[]  KtParamMax=[]  KbOutMin=[]  KbOutMax=[]  KtOutMin=[]  KtOutMax=[]  IntegratorOutMin=[]  IntegratorOutMax=[]  FilterOutMin=[]  FilterOutMax=[]  SumI1OutMin=[]  SumI1OutMax=[]  SumI2OutMin=[]  SumI2OutMax=[]  SumI3OutMin=[]  SumI3OutMax=[]  SumI4OutMin=[]  SumI4OutMax=[]  SumDOutMin=[]  SumDOutMax=[]  DifferentiatorOutMin=[]  DifferentiatorOutMax=[]  FilterDiffOutCoefMin=[]  FilterDiffOutCoefMax=[]  ReciprocalOutMin=[]  ReciprocalOutMax=[]  SumDenOutMin=[]  SumDenOutMax=[]  SumNumOutMin=[]  SumNumOutMax=[]  DivideOutMin=[]  DivideOutMax=[]  UdiffTsProdOutMin=[]  UdiffTsProdOutMax=[]  NTsProdOutMin=[]  NTsProdOutMax=[]  UintegralTsProdOutMin=[]  UintegralTsProdOutMax=[]  UngainTsProdOutMin=[]  UngainTsProdOutMax=[]  IntegratorContinuousStateAttributes=''  IntegratorStateMustResolveToSignalObject=off  IntegratorRTWStateStorageClass=Auto  FilterContinuousStateAttributes=''  FilterStateMustResolveToSignalObject=off  FilterRTWStateStorageClass=Auto  ParallelPVariant=ExternalParameters  IdealPVariant=Disabled  IVariant=ExternalParameters  DVariant=Disabled  IntegratorVariant=Discrete  SatVariant=Enabled  AWVariant=DiscClampingParallel  PCopyVariant=Disabled  TRVariant=Disabled  FdbkBlocksVariant=Forward  IdealPFdbkVariant=Disabled  SatFdbkVariant=Disabled  DerivativeFilterVariant=Disabled  NVariant=Disabled  NCopyVariant=Disabled_SignalSpec  FilterICVariant=Disabled  IntegratorICVariant=InternalICs  ExternalResetVariant=Disabled  TRSumVariant=Passthrough  SumFdbkVariant=Disabled  SumVariant=Sum_PI  TsampFilterVariant=InternalTs  TsampNgainVariant=Passthrough  TsampIntegralVariant=Passthrough  ExternalSaturationOutDataTypeStr=Inherit: Same as second input
  Product1 : Product
  Product2 : Product
  Scope : Scope  NumInputPorts=2
  Sine_Cosine : Subsystem  TreatAsAtomicUnit=on
      settings: RTWSystemCode=Nonreusable function  RTWFcnNameOpts=Use subsystem name
  SpeedToTheta : Subsystem
  Subsystem1 : Subsystem
  Sum : Sum  Inputs=|--
  Unit Delay : UnitDelay  SampleTime=-1  HasFrameUpgradeWarning=on
  Theta : Outport
  speed_hat : Outport  Port=2
  wires:
  Sine_Cosine/2(Sin) -> Product1/2
  Subsystem1/1(Out) -> PIDTheta_Ctrl/1
  Sine_Cosine/1(Cos) -> Product2/1
  Sum/1 -> Subsystem1/1(Err_in)
  Product1/1 -> Sum/2
  Product2/1 -> Sum/1
  e_beta_hat/1 -> Scope/2, Product1/1
  e_alpha_hat/1 -> Scope/1, Product2/2
  Unit Delay/1 -> Subsystem1/2(speed), speed_hat/1  "speed_hat"
  SpeedToTheta/1(Out1) -> [theta_hat]  "ObserverTheta"
  PIDTheta_Ctrl/1 -> SpeedToTheta/1(In1), Unit Delay/1
  [theta_hat] -> Theta/1
  Kp/1 -> PIDTheta_Ctrl/2
  Ki/1 -> PIDTheta_Ctrl/3
  [theta_hat] -> Sine_Cosine/1(P)

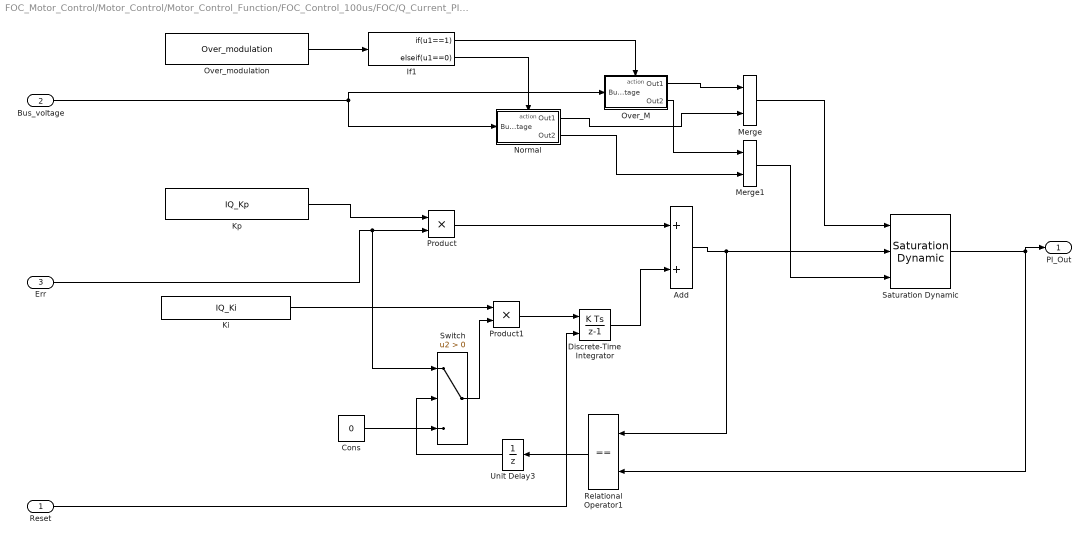
== system FOC_Motor_Control/Motor_Control/Motor_Control_Function/FOC_Control_100us/FOC/Q_Current_PI/IQ_Control ==
  Reset : Inport
  Bus_voltage : Inport  Port=2
  Err : Inport  Port=3
  Add : Sum
  Cons : Constant  Value=0  OutDataTypeStr=single
  Discrete-Time Integrator : DiscreteIntegrator  ExternalReset=level  SampleTime=-1  ICPrevOutput=DiscIntNeverNeededParam  ICPrevScaledInput=DiscIntNeverNeededParam
  If1 : If  IfExpression=u1==1  ElseIfExpressions=u1==0  ShowElse=off
  Ki : Constant  Value=IQ_Ki  OutDataTypeStr=single
  Kp : Constant  Value=IQ_Kp  OutDataTypeStr=single
  Merge : Merge
  Merge1 : Merge
  Normal : Subsystem  TreatAsAtomicUnit=on
  Over_M : Subsystem  TreatAsAtomicUnit=on
  Over_modulation : Constant  Value=Over_modulation  OutDataTypeStr=boolean
  Product : Product
  Product1 : Product
  Relational Operator1 : RelationalOperator  Operator===  OutDataTypeStr=boolean  RndMeth=Simplest
  Saturation Dynamic : simulink/Discontinuities/Saturation Dynamic  OutMin=[]  OutMax=[]  OutDataTypeStr=Inherit: Same as second input  OutDataType=fixdt(1, 16)  OutScaling=2^-10  DoSatur=off
  Switch : Switch  Criteria=u2 > Threshold
  Unit Delay3 : UnitDelay  SampleTime=-1  HasFrameUpgradeWarning=on
  PI_Out : Outport
  wires:
  Kp/1 -> Product/1
  Err/1 -> Switch/1, Product/2
  Switch/1 -> Product1/2
  Product1/1 -> Discrete-Time Integrator/1
  Product/1 -> Add/1
  Add/1 -> Saturation Dynamic/2, Relational Operator1/1
  Saturation Dynamic/1 -> PI_Out/1, Relational Operator1/2
  Cons/1 -> Switch/3
  Discrete-Time Integrator/1 -> Add/2
  Relational Operator1/1 -> Unit Delay3/1
  Ki/1 -> Product1/1
  Unit Delay3/1 -> Switch/2
  Reset/1 -> Discrete-Time Integrator/2
  Normal/1(Out1) -> Merge/2
  Over_M/1(Out1) -> Merge/1
  Over_modulation/1 -> If1/1
  Normal/2(Out2) -> Merge1/2
  If1/2 -> Normal/Action
  Bus_voltage/1 -> Normal/1(Bus_voltage), Over_M/1(Bus_voltage)
  If1/1 -> Over_M/Action
  Over_M/2(Out2) -> Merge1/1
  Merge/1 -> Saturation Dynamic/1
  Merge1/1 -> Saturation Dynamic/3

== system FOC_Motor_Control/Motor_Control/Motor_Control_Function/FOC_Control_100us/FOC/SVPWM/Disable_Motor ==
  Action Port : ActionPort  ActionPortLabel=elseif(u1==1)
  Constant : Constant  Value=0  OutDataTypeStr=single
  Constant1 : Constant  Value=0  OutDataTypeStr=single
  Constant2 : Constant  Value=0  OutDataTypeStr=single
  Out1 : Outport
  Out2 : Outport  Port=2
  Out3 : Outport  Port=3
  wires:
  Constant/1 -> Out1/1
  Constant1/1 -> Out2/1
  Constant2/1 -> Out3/1

== system FOC_Motor_Control/Motor_Control/Motor_Control_Function/FOC_Control_100us/FOC/SVPWM/Enable_Motor ==
  In1 : Inport
  In2 : Inport  Port=2
  In3 : Inport  Port=3
  Action Port : ActionPort  ActionPortLabel=if(u1==0)
  Saturation : Saturate  UpperLimit=4199  LowerLimit=1
  Saturation1 : Saturate  UpperLimit=4199  LowerLimit=1
  Saturation2 : Saturate  UpperLimit=4199  LowerLimit=1
  Out1 : Outport
  Out2 : Outport  Port=2
  Out3 : Outport  Port=3
  wires:
  In1/1 -> Saturation/1
  In2/1 -> Saturation1/1
  In3/1 -> Saturation2/1
  Saturation/1 -> Out1/1
  Saturation1/1 -> Out2/1
  Saturation2/1 -> Out3/1

== system FOC_Motor_Control/Motor_Control/Motor_Control_Function/FOC_Control_100us/FOC/SVPWM/N Sector  Caculate ==
  Ubelta : Inport
  Ualf : Inport  Port=2
  Add : Sum  Inputs=+++
  Add1 : Sum  Inputs=-+  OutDataTypeStr=single
  Add2 : Sum  Inputs=--  OutDataTypeStr=single
  Constant : Constant  OutDataTypeStr=single
  Constant1 : Constant  Value=0  OutDataTypeStr=single
  Gain : Gain  Gain=sqrt(3)
  Gain1 : Gain  Gain=2
  Gain2 : Gain  Gain=4
  Saturation : Saturate  UpperLimit=6  LowerLimit=1
  Switch : Switch
  Switch1 : Switch
  Switch2 : Switch
  N : Outport
  wires:
  Saturation/1 -> N/1
  Add/1 -> Saturation/1
  Gain2/1 -> Add/3
  Switch2/1 -> Gain2/1
  Add2/1 -> Switch2/2
  Gain1/1 -> Add/2
  Switch1/1 -> Gain1/1
  Add1/1 -> Switch1/2
  Gain/1 -> Add2/2, Add1/2
  Ualf/1 -> Gain/1
  Switch/1 -> Add/1
  Constant1/1 -> Switch/3, Switch1/3, Switch2/3
  Constant/1 -> Switch/1, Switch1/1, Switch2/1
  Ubelta/1 -> Add2/1, Add1/1, Switch/2

== system FOC_Motor_Control/Motor_Control/Motor_Control_Function/FOC_Control_100us/FOC/SVPWM/T1 T2  Caculate ==
  note: Z
  note: Y
  note: -X
  note: X
  note: -Y
  note: Y
  note: -X
  note: X
  note: Z
  note: -Y
  note: -Z
  note: X
  note: Y
  note: Z
  N : Inport
  X : Inport  Port=2
  Y : Inport  Port=3
  Z : Inport  Port=4
  Tpwm : Inport  Port=5
  Add : Sum
  Add1 : Sum  Inputs=-+
  Divide : Product  Inputs=**/
  Divide1 : Product  Inputs=/**
  Gain : Gain  Gain=-1
  Gain1 : Gain  Gain=-1
  Gain2 : Gain  Gain=-1
  Index Vector : MultiPortSwitch  Inputs=6
  Index Vector1 : MultiPortSwitch  Inputs=6
  Switch : Switch  Criteria=u2 > Threshold
  Switch2 : Switch  Criteria=u2 > Threshold
  T1 : Outport
  T2 : Outport  Port=2
  wires:
  Switch2/1 -> T2/1
  Divide1/1 -> Switch2/3
  Switch/1 -> T1/1
  Add1/1 -> Switch/2, Switch2/2
  Add/1 -> Divide1/1, Divide/3, Add1/1
  Tpwm/1 -> Divide1/2, Divide/2, Add1/2
  Divide/1 -> Switch/3
  Index Vector1/1 -> Switch2/1, Add/2, Divide1/3
  Index Vector/1 -> Switch/1, Divide/1, Add/1
  Gain1/1 -> Index Vector/7, Index Vector1/6
  Gain2/1 -> Index Vector/4, Index Vector1/7  "-Z"
  Gain/1 -> Index Vector/5, Index Vector1/3
  Y/1 -> Gain1/1, Index Vector/3, Index Vector1/2
  X/1 -> Index Vector1/4, Index Vector/6, Gain/1
  Z/1 -> Index Vector/2, Index Vector1/5, Gain2/1
  N/1 -> Index Vector1/1, Index Vector/1
